simulink model "pitch_control_sim"  (R2020a)
settings: Solver=VariableStepAuto  StartTime=0.0  StopTime=400  RelTol=1e-3
undefined symbols (not defined in the file): den, num
settings Model: Creator=lum  LastModifiedBy=lum

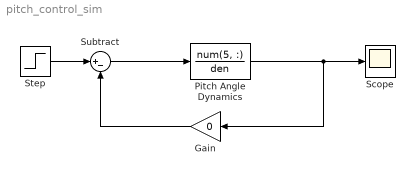
== system pitch_control_sim ==
  Gain : Gain  Gain=0
  Pitch Angle Dynamics : TransferFcn  Numerator=num(5, :)  Denominator=den  ContinuousStateAttributes='pitch_angle'
  Scope : Scope
  Step : Step  Time=0  After=deg2rad(1)  SampleTime=0
  Subtract : Sum  Inputs=|+-
  wires:
  Pitch Angle Dynamics/1 -> Gain/1, Scope/1
  Gain/1 -> Subtract/2
  Step/1 -> Subtract/1
  Subtract/1 -> Pitch Angle Dynamics/1
